simulink model "parallel_fp"  (R2021a)
settings: Solver=VariableStepAuto  StartTime=0.0  StopTime=5  RelTol=1e-3
values from neighbouring files (symbols this model uses):
  k_fi = 1.5*eye(3)    [params.m]
  k_fp = 0.5*eye(3)    [params.m]
  kd = 2*z*w    [params.m]
  kp = w^2    [params.m]
  Md = 0.4*diag([1 1 1])    [params.m]
settings Model: Creator=Sebastiano  LastModifiedBy=antoninoparisi
settings SolverCC: AlgebraicLoopSolver=TrustRegion
settings DebuggingCC: SFMachineParentedDataDiag=warning

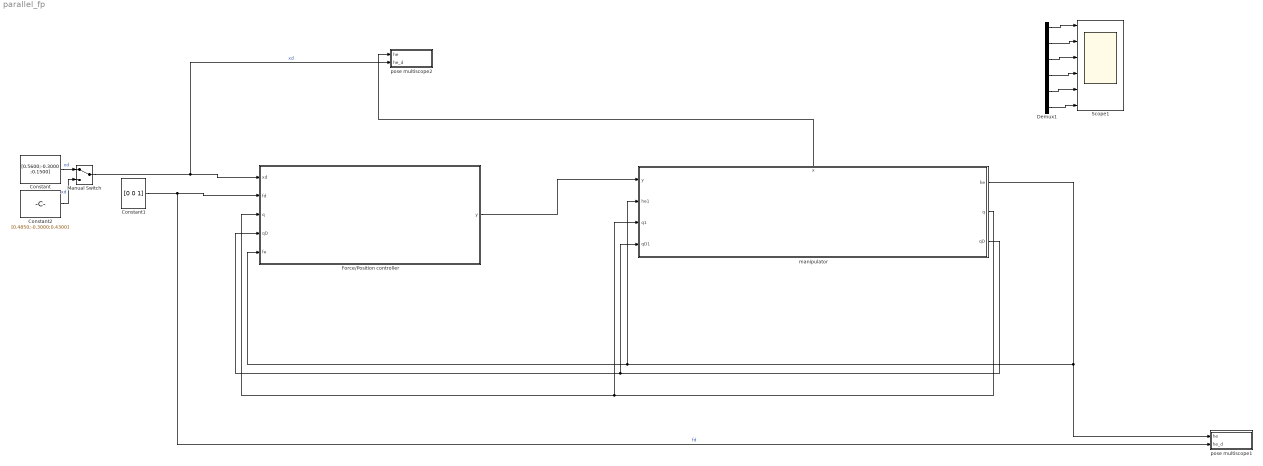
== system parallel_fp ==
  Constant : Constant  Value=|  VectorParams1D=off
      | [0.5600;-0.3000
      |  ;0.1500]
  Constant1 : Constant  Value=[0 0 1]  VectorParams1D=off
  Constant2 : Constant  Value=[0.4850;-0.3000;0.4300]  VectorParams1D=off
  Demux1 : Demux  Outputs=6
  Force/Position controller : Subsystem
  Manual Switch : ManualSwitch
  Scope1 : Scope  NumInputPorts=6
  manipulator : Subsystem
      settings: PortSchema="{\"entries\":[{\"content\":{\"sides\":[{\"content\":{\"connectorIds\":[\"In1\",\"In2\",\"In3\",\"In4\"]},\"type\":\"ConnectorPlacement.EquallySpacedRectSide\",\"uuid\":\"45511188-ca76-4924-8a71-b5f2f17f909c\"},{\"content\":{\"connectorIds\":[\"Out1\",\"Out2\",\"Out3\"],\"side\":\"RIGHT\"},\"type\":\"ConnectorPlacement.EquallySpacedRectSide\",\"uuid\":\"d337272a-4a73-4c76-919a-8b9784c4210c\"},{\"content\":{\"connectorIds\":[\"Out4\"],\"side\":\"TOP\"},\"type\":\"ConnectorPlacement.EquallySpacedRectSide\",\"uuid\":\"0c2f2d5e-17ee-42eb-b5f4-ba35f78be37b\"}]},\"type\":\"ConnectorPlacement.EquallySpacedConnector\",\"uuid\":\"e35002c1-7fa0-44ea-9880-068f21661f1d\"}],\"packageUris\":[\"http://schema.mathworks.com/mf0/Connector/R2020b\"],\"version\":\"1.0\"}"
  pose multiscope1 : Subsystem
  pose multiscope2 : Subsystem
  wires:
  Constant1/1 -> pose multiscope1/2(he_d), Force/Position controller/2(fd)  "fd"
  Manual Switch/1 -> pose multiscope2/2(he_d), Force/Position controller/1(xd)  "xd"
  Force/Position controller/1(y) -> manipulator/1(y)
  manipulator/2(q) -> manipulator/3(q1), Force/Position controller/3(q)
  manipulator/3(qD) -> manipulator/4(qD1), Force/Position controller/4(qD)
  manipulator/1(he) -> pose multiscope1/1(he), Force/Position controller/5(fe), manipulator/2(he1)
  Demux1/5 -> Scope1/5
  Demux1/1 -> Scope1/1
  Demux1/2 -> Scope1/2
  Demux1/6 -> Scope1/6
  Demux1/3 -> Scope1/3
  Demux1/4 -> Scope1/4
  manipulator/4(x) -> pose multiscope2/1(he)
  Constant/1 -> Manual Switch/1  "xd"
  Constant2/1 -> Manual Switch/2  "xd"

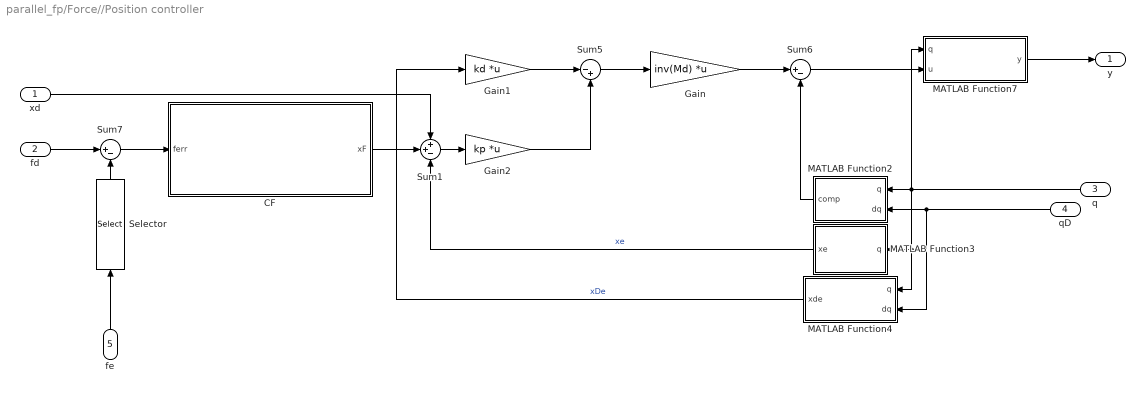
== system parallel_fp/Force//Position controller ==
  xd : Inport
  fd : Inport  Port=2
  q : Inport  Port=3
  qD : Inport  Port=4
  fe : Inport  Port=5
  CF : Subsystem
  Gain : Gain  Gain=inv(Md)  Multiplication=Matrix(K*u) (u vector)
  Gain1 : Gain  Gain=kd  Multiplication=Matrix(K*u) (u vector)
  Gain2 : Gain  Gain=kp  Multiplication=Matrix(K*u) (u vector)
  MATLAB Function2 : MATLAB Function  TreatAsAtomicUnit=on
  MATLAB Function3 : MATLAB Function  TreatAsAtomicUnit=on
  MATLAB Function4 : MATLAB Function  TreatAsAtomicUnit=on
  MATLAB Function7 : MATLAB Function  TreatAsAtomicUnit=on
  Selector : Selector  InputPortWidth=6  IndexOptions=Starting index (dialog)  Indices=1  OutputSizes=3
  Sum1 : Sum  Inputs=++-
  Sum5 : Sum  Inputs=|-+
  Sum6 : Sum  Inputs=|+-
  Sum7 : Sum  Inputs=|+-
  y : Outport
  wires:
  fd/1 -> Sum7/1
  Sum1/1 -> Gain2/1
  Gain/1 -> Sum6/1
  MATLAB Function4/1(xde) -> Gain1/1  "xDe"
  Gain1/1 -> Sum5/1
  Sum5/1 -> Gain/1
  MATLAB Function2/1(comp) -> Sum6/2
  Sum6/1 -> MATLAB Function7/2(u)
  MATLAB Function3/1(xe) -> Sum1/3  "xe"
  Gain2/1 -> Sum5/2
  MATLAB Function7/1(y) -> y/1
  qD/1 -> MATLAB Function4/2(dq), MATLAB Function2/2(dq)
  q/1 -> MATLAB Function7/1(q), MATLAB Function2/1(q), MATLAB Function4/1(q), MATLAB Function3/1(q)
  Sum7/1 -> CF/1(ferr)
  CF/1(xF) -> Sum1/2
  xd/1 -> Sum1/1
  fe/1 -> Selector/1
  Selector/1 -> Sum7/2

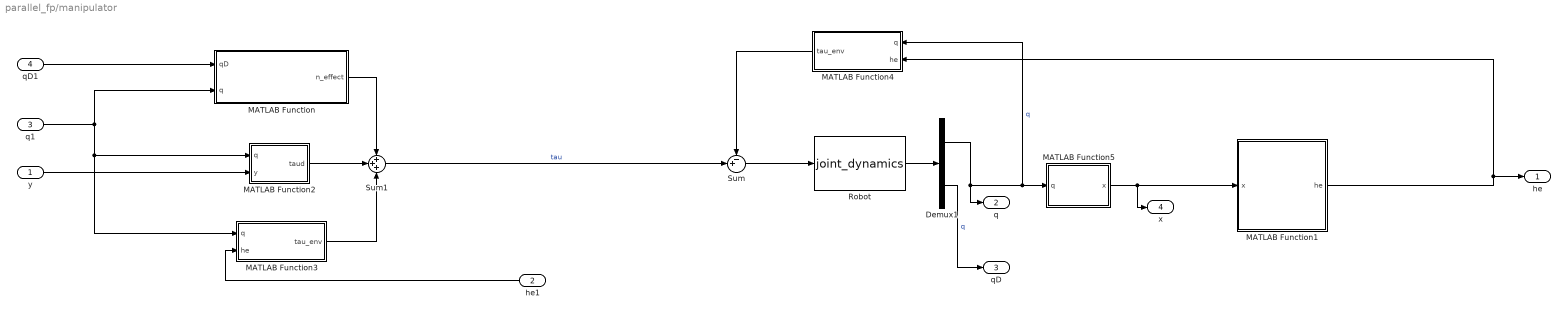
== system parallel_fp/manipulator ==
  y : Inport
  he1 : Inport  Port=2
  q1 : Inport  Port=3
  qD1 : Inport  Port=4
  Demux1 : Demux  Outputs=[3, 3]
  MATLAB Function : MATLAB Function  TreatAsAtomicUnit=on
  MATLAB Function1 : MATLAB Function  TreatAsAtomicUnit=on
  MATLAB Function2 : MATLAB Function  TreatAsAtomicUnit=on
  MATLAB Function3 : MATLAB Function  TreatAsAtomicUnit=on
  MATLAB Function4 : MATLAB Function  TreatAsAtomicUnit=on
  MATLAB Function5 : MATLAB Function  TreatAsAtomicUnit=on
  Robot : S-Function  FunctionName=joint_dynamics  Parameters=robot  SFunctionDeploymentMode=off  EnableBusSupport=off
  Sum : Sum  Inputs=-+|
  Sum1 : Sum  Inputs=+++
  he : Outport
  q : Outport  Port=2
  qD : Outport  Port=3
  x : Outport  Port=4
  wires:
  Sum/1 -> Robot/1
  Robot/1 -> Demux1/1
  MATLAB Function4/1(tau_env) -> Sum/1
  MATLAB Function5/1(x) -> x/1, MATLAB Function1/1(x)
  MATLAB Function1/1(he) -> MATLAB Function4/2(he), he/1
  Demux1/1 -> MATLAB Function5/1(q), MATLAB Function4/1(q), q/1  "q"
  he1/1 -> MATLAB Function3/2(he)
  qD1/1 -> MATLAB Function/1(qD)
  y/1 -> MATLAB Function2/2(y)
  MATLAB Function/1(n_effect) -> Sum1/1
  Sum1/1 -> Sum/2  "tau"
  q1/1 -> MATLAB Function/2(q), MATLAB Function3/1(q), MATLAB Function2/1(q)
  MATLAB Function3/1(tau_env) -> Sum1/3
  MATLAB Function2/1(taud) -> Sum1/2
  Demux1/2 -> qD/1  "q"

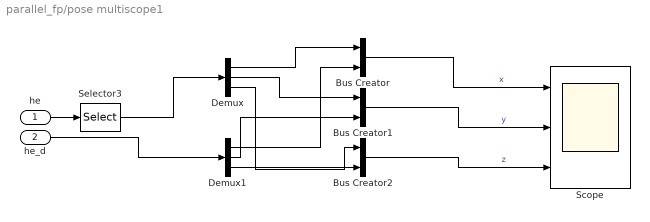
== system parallel_fp/pose multiscope1 ==
  he : Inport
  he_d : Inport  Port=2
  Bus Creator : BusCreator  Inputs=2
  Bus Creator1 : BusCreator  Inputs=2
  Bus Creator2 : BusCreator  Inputs=2
  Demux : Demux  Outputs=3
  Demux1 : Demux  Outputs=3
  Scope : Scope  NumInputPorts=3
  Selector3 : Selector  InputPortWidth=6  IndexOptions=Starting index (dialog)  Indices=1  OutputSizes=3
  wires:
  he_d/1 -> Demux1/1
  he/1 -> Selector3/1
  Selector3/1 -> Demux/1
  Demux/1 -> Bus Creator/1
  Demux1/1 -> Bus Creator/2
  Demux/2 -> Bus Creator1/1
  Demux/3 -> Bus Creator2/1
  Demux1/2 -> Bus Creator1/2
  Demux1/3 -> Bus Creator2/2
  Bus Creator/1 -> Scope/1  "x"
  Bus Creator1/1 -> Scope/2  "y"
  Bus Creator2/1 -> Scope/3  "z"

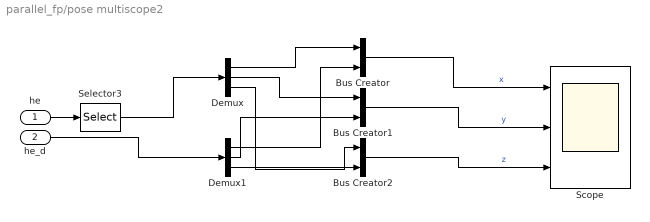
== system parallel_fp/pose multiscope2 ==
  he : Inport
  he_d : Inport  Port=2
  Bus Creator : BusCreator  Inputs=2
  Bus Creator1 : BusCreator  Inputs=2
  Bus Creator2 : BusCreator  Inputs=2
  Demux : Demux  Outputs=3
  Demux1 : Demux  Outputs=3
  Scope : Scope  NumInputPorts=3
  Selector3 : Selector  InputPortWidth=6  IndexOptions=Starting index (dialog)  Indices=1  OutputSizes=3
  wires:
  he_d/1 -> Demux1/1
  he/1 -> Selector3/1
  Selector3/1 -> Demux/1
  Demux/1 -> Bus Creator/1
  Demux1/1 -> Bus Creator/2
  Demux/2 -> Bus Creator1/1
  Demux/3 -> Bus Creator2/1
  Demux1/2 -> Bus Creator1/2
  Demux1/3 -> Bus Creator2/2
  Bus Creator/1 -> Scope/1  "x"
  Bus Creator1/1 -> Scope/2  "y"
  Bus Creator2/1 -> Scope/3  "z"

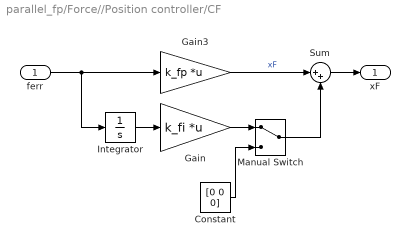
== system parallel_fp/Force//Position controller/CF ==
  ferr : Inport
  Constant : Constant  Value=[0 0 0]
  Gain : Gain  Gain=k_fi  Multiplication=Matrix(K*u) (u vector)
  Gain3 : Gain  Gain=k_fp  Multiplication=Matrix(K*u) (u vector)
  Integrator : Integrator
  Manual Switch : ManualSwitch
  Sum : Sum  Inputs=|++
  xF : Outport
  wires:
  ferr/1 -> Integrator/1, Gain3/1
  Gain3/1 -> Sum/1  "xF"
  Sum/1 -> xF/1
  Gain/1 -> Manual Switch/1
  Manual Switch/1 -> Sum/2
  Integrator/1 -> Gain/1
  Constant/1 -> Manual Switch/2

== matlab function parallel_fp/Force//Position controller/MATLAB Function2 ==
  data: q input; comp output; dq input
function comp = JpD(q, dq)

   
Jpd = jacobian_dot(q,dq);

Jpd = Jpd(1:3,:);

comp = Jpd*dq;

== matlab function parallel_fp/Force//Position controller/MATLAB Function3 ==
  data: q input; xe output
function xe = Kp(q)

t1 = q(1);
d1 = q(2);
t2 = q(3);


a1 = 0.15;
a2 = 0.4;
a3 = 0.3;
a4 = 0.16;


K = [[cos(t1)*cos(t2), -cos(t1)*sin(t2), -sin(t1),      a2*cos(t1) + a4*cos(t1)*cos(t2)]
    [        sin(t2),          cos(t2),        0,                 a4*sin(t2) - d1 - a3]
    [cos(t2)*sin(t1), -sin(t1)*sin(t2),  cos(t1), a1 + a2*sin(t1) + a4*cos(t2)*sin(t1)]
    [              0,                0,        0,                                    1]];

xe = K(1:3, 4);

== matlab function parallel_fp/Force//Position controller/MATLAB Function4 ==
  data: q input; xde output; dq input
function xde = Jp(q, dq)

J = jacobian(q);
Jp = J(1:3,:);
xde = Jp * dq;

== matlab function parallel_fp/Force//Position controller/MATLAB Function7 ==
  data: q input; u input; y output
function y = Jpinv(q, u)

J = jacobian(q);
Jp = J(1:3,:);
y =  pinv(Jp) * u;

== matlab function parallel_fp/manipulator/MATLAB Function ==
  data: qD input; q input; n_effect output
function n_effect = n(qD, q)

n_effect = C_Lagrangian(q, qD)*qD + G_Lagrangian(q);

== matlab function parallel_fp/manipulator/MATLAB Function1 ==
  data: x input; he output
function he = environment(x)

% environment params
K = diag([15 15 15 0.1 0.1 0.1]);    % stiffness
wall = 0.4; % constraint position w.r.t. frame 0 (it's y=-0.5 w.r.t. base frame)

if x(3) >= wall  % check is done in frame 0
    xr = x;
    xr(3) = wall;
    % calculate the forces
    x_diff = x - xr;
    he = K * x_diff;
else
    % free motion
    he = zeros(6,1);
end

== matlab function parallel_fp/manipulator/MATLAB Function2 ==
  data: q input; taud output; y input
function taud = B(q, y)

taud = B_Lagrangian(q)*y;

== matlab function parallel_fp/manipulator/MATLAB Function3 ==
  data: q input; he input; tau_env output
function tau_env = J(q, he)

tau_env = jacobian(q)' * he;

== matlab function parallel_fp/manipulator/MATLAB Function4 ==
  data: q input; he input; tau_env output
function tau_env = J(q, he)

tau_env = jacobian(q)' * he;

== matlab function parallel_fp/manipulator/MATLAB Function5 ==
  data: q input; x output
function x = K(q)

t1 = q(1);
d1 = q(2);
t2 = q(3);


a1 = 0.15;
a2 = 0.4;
a3 = 0.3;
a4 = 0.16;


% wrt frame 0
K = [[cos(t1)*cos(t2), -cos(t1)*sin(t2), -sin(t1),      a2*cos(t1) + a4*cos(t1)*cos(t2)]
    [        sin(t2),          cos(t2),        0,                 a4*sin(t2) - d1 - a3]
    [cos(t2)*sin(t1), -sin(t1)*sin(t2),  cos(t1), a1 + a2*sin(t1) + a4*cos(t2)*sin(t1)]
    [              0,                0,        0,                                    1]];

pos = K(1:3, 4);
ori = rotm2eul(K(1:3,1:3), 'ZYZ')';

x = [pos; ori];
